simulink model "HW_1_v2_2019a_subsystem"  (R2019a)
settings: Solver=VariableStepAuto  StartTime=0.0  StopTime=70  RelTol=1e-12
model workspace (MAT data in the model file):
  d_tar = 20
values from neighbouring files (symbols this model uses):
  d_0 = 8    [acc1.m]
  t_H_tar = 1    [acc1.m]
  v_H0 = 28    [acc1.m]
  v_L0 = 36    [acc1.m]
  v_tar = 36    [acc1.m]
  x_H0 = 0    [acc1.m]
  x_L0 = 50    [acc1.m]
undefined symbols (not defined in the file or in its folder): sigbuilder_block
libraries: cstblocks x3
settings Model: Creator=jake  LastModifiedBy=andreasjonsson
settings DebuggingCC: SFMachineParentedDataDiag=error

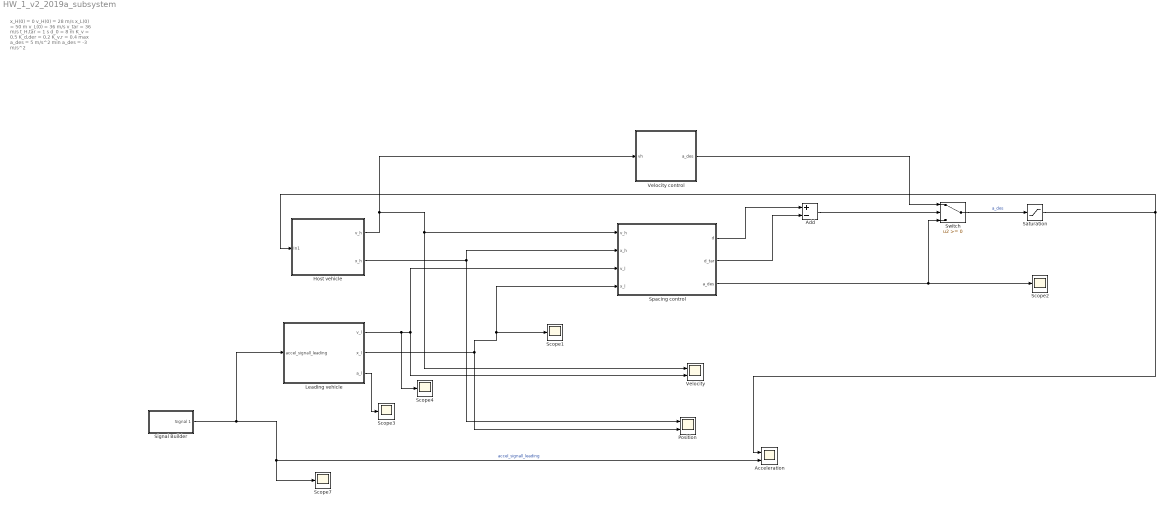
== system HW_1_v2_2019a_subsystem ==
  note: x_H(0) = 0
      | v_H(0) = 28 m/s
      |
      | x_L(0) = 50 m
      | v_L(0) = 36 m/s
      |
      | v_tar = 36 m/s
      | t_H,tar = 1 s
      | d_0 = 8 m
      |
      | K_v = 0.5
      | K_d,der = 0.2
      | K_v,r = 0.4
      |
      | max a_des = 5 m/s^2
      | min a_des = -3 m/s^2
  Acceleration : Scope  NumInputPorts=2
  Add : Sum  Inputs=+-
  Host vehicle : Subsystem
  Leading vehicle : Subsystem
  Position : Scope  NumInputPorts=2
  Saturation : Saturate  UpperLimit=5  LowerLimit=-3
  Scope{1..4,7} (5 alike) : Scope
  Signal Builder : Subsystem  Tag=STV Subsys  LoadFcn=sigbuilder_block('load');  StartFcn=sigbuilder_block('start');  StopFcn=sigbuilder_block('stop');  ClipboardFcn=sigbuilder_block('clipboard');  mask(Sigbuilder block){tuvar=[0:10]}
      mask help: Simulink:masks:SigbuilderBlock_MD
      mask init:
      | if ~strcmp(get_param(bdroot(gcbh),'SimulationStatus'),'stopped') tuvar = sigbuilder_block('maskInit'); end
      settings: CopyFcn=sigbuilder_block('copy');  DeleteFcn=sigbuilder_block('delete');  ModelCloseFcn=sigbuilder_block('modelClose');  PreSaveFcn=sigbuilder_block('preSave');  PauseFcn=sigbuilder_block('pause');  ContinueFcn=sigbuilder_block('continue');  NameChangeFcn=sigbuilder_block('namechange');  OpenFcn=sigbuilder_block('open',[553.5 167.25 843.75 498.75 ]);  CloseFcn=sigbuilder_block('close');
      mask Display: plot(0, 0, 100, 100,[2, 2, 32, 32, 2], [68, 8, 8, 68, 68],[32, 2], [38, 38], [32, 19, 2],[53, 60, 44], [32, 17, 17, 2],[16, 16, 31, 31]);txt = getActiveGroup(gcbh);text(2, 100, txt,'verticalAlignment', 'top');
  Spacing control : Subsystem
  Switch : Switch
  Velocity : Scope  NumInputPorts=2
  Velocity control : Subsystem
  wires:
  Switch/1 -> Saturation/1  "a_des"
  Signal Builder/1(Signal 1) -> Leading vehicle/1(accel_signall_leading), Scope7/1, Acceleration/2  "accel_signall_leading"
  Saturation/1 -> Host vehicle/1(In1), Acceleration/1
  Add/1 -> Switch/2
  Host vehicle/1(v_h) -> Velocity control/1(vh), Velocity/1, Spacing control/1(v_h)
  Host vehicle/2(x_h) -> Spacing control/2(x_h), Position/1
  Leading vehicle/1(v_l) -> Spacing control/3(v_l), Velocity/2, Scope4/1
  Leading vehicle/2(x_l) -> Spacing control/4(x_l), Scope1/1, Position/2
  Leading vehicle/3(a_l) -> Scope3/1
  Velocity control/1(a_des) -> Switch/1
  Spacing control/3(a_des) -> Scope2/1, Switch/3
  Spacing control/1(d) -> Add/1
  Spacing control/2(d_tar) -> Add/2

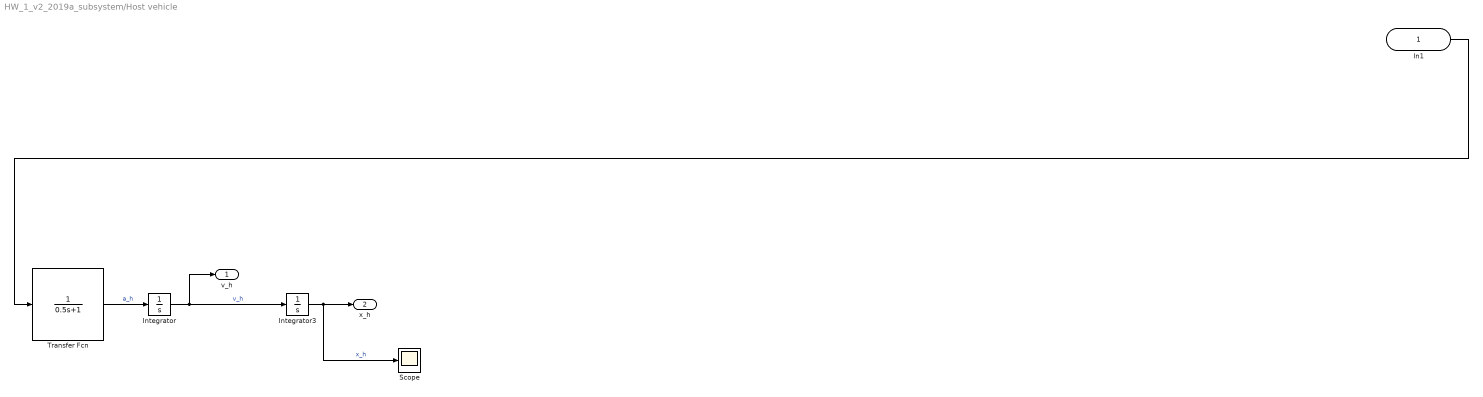
== system HW_1_v2_2019a_subsystem/Host vehicle ==
  In1 : Inport
  Integrator : Integrator  InitialCondition=v_H0
  Integrator3 : Integrator  InitialCondition=x_H0
  Scope : Scope
  Transfer Fcn : TransferFcn  Denominator=[0.5 1]
  v_h : Outport
  x_h : Outport  Port=2
  wires:
  Integrator/1 -> Integrator3/1, v_h/1  "v_h"
  Transfer Fcn/1 -> Integrator/1  "a_h"
  In1/1 -> Transfer Fcn/1
  Integrator3/1 -> Scope/1, x_h/1  "x_h"

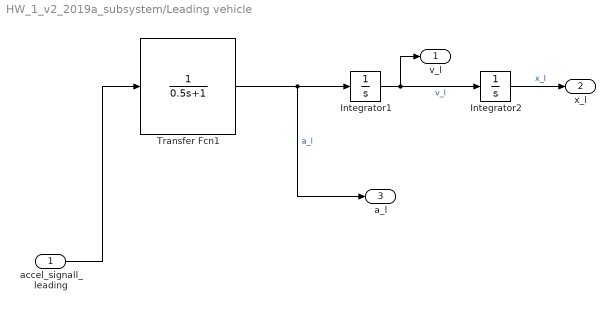
== system HW_1_v2_2019a_subsystem/Leading vehicle ==
  accel_signall_leading : Inport
  Integrator1 : Integrator  InitialCondition=v_L0
  Integrator2 : Integrator  InitialCondition=x_L0
  Transfer Fcn1 : TransferFcn  Denominator=[0.5 1]
  v_l : Outport
  x_l : Outport  Port=2
  a_l : Outport  Port=3
  wires:
  Integrator2/1 -> x_l/1  "x_l"
  accel_signall_leading/1 -> Transfer Fcn1/1
  Integrator1/1 -> Integrator2/1, v_l/1  "v_l"
  Transfer Fcn1/1 -> a_l/1, Integrator1/1  "a_l"

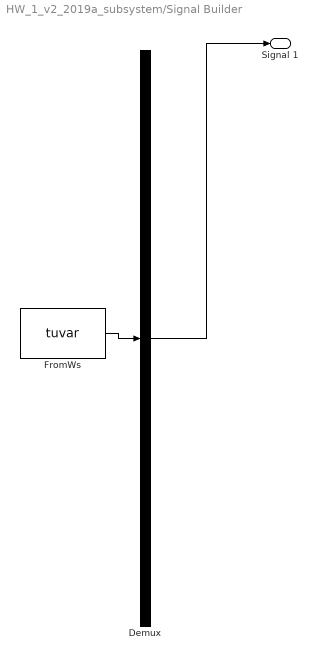
== system HW_1_v2_2019a_subsystem/Signal Builder ==
  Demux : Demux  Tag=STV Demux  Outputs=1
  FromWs : FromWorkspace  Tag=STV FromWs  VariableName=tuvar  SampleTime=0
      SigBuilderData=|
      | common.afterFinalStr = 'Extrapolate'
      | common.sampleTime = 0
      | dataSet.timeRange = [0 46]
      | dataSet.name = 'Group 1'
      | sbobj.Groups.Name = 'Group 1'
      | sbobj.Groups.Signals.Name = 'Signal 1'
      | sbobj.Groups.Signals.XData = [0 10 10.5 13.5 14 40 40.5 43.5 44 46]
      | sbobj.Groups.Signals.YData = [0 0 -2 -2 0 0 2 2 0 0.02]
      | sbobj.Groups.TimeRange = [0 46]
  Signal 1 : Outport  Tag=STV Outport  VectorParamsAs1DForOutWhenUnconnected=on
  wires:
  Demux/1 -> Signal 1/1
  FromWs/1 -> Demux/1

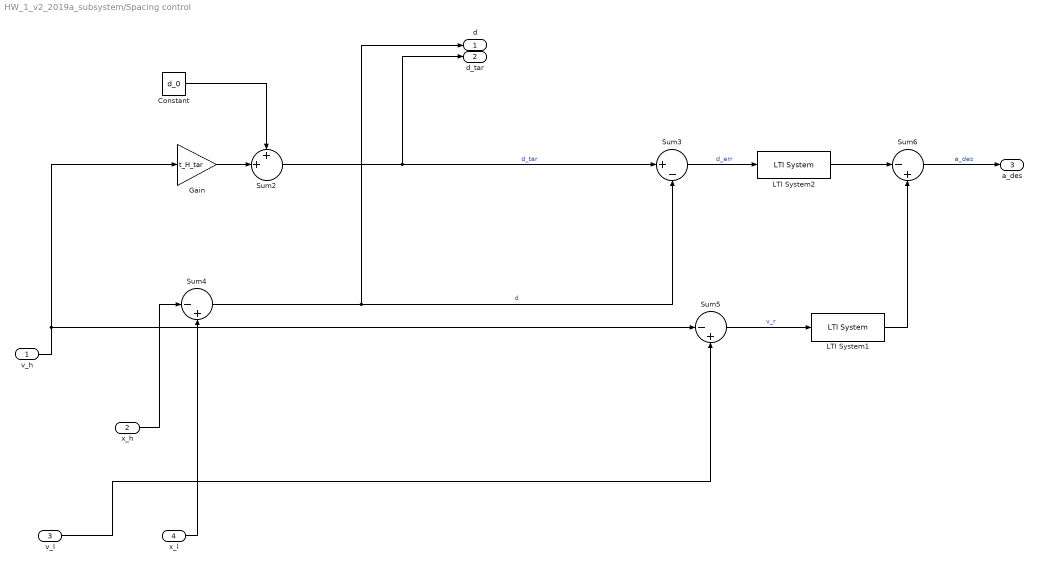
== system HW_1_v2_2019a_subsystem/Spacing control ==
  v_h : Inport
  x_h : Inport  Port=2
  v_l : Inport  Port=3
  x_l : Inport  Port=4
  Constant : Constant  Value=d_0
  Gain : Gain  Gain=t_H_tar
  LTI System1 : cstblocks/LTI System  sys=K_v_r  IC=[]
  LTI System2 : cstblocks/LTI System  sys=K_d_err  IC=[]
  Sum2 : Sum  Inputs=++|
  Sum3 : Sum  Inputs=|+-
  Sum4 : Sum  Inputs=|-+
  Sum5 : Sum  Inputs=|-+
  Sum6 : Sum  Inputs=|-+
  d : Outport
  d_tar : Outport  Port=2
  a_des : Outport  Port=3
  wires:
  x_l/1 -> Sum4/2
  v_l/1 -> Sum5/2
  Sum6/1 -> a_des/1  "a_des"
  Sum4/1 -> d/1, Sum3/2  "d"
  LTI System1/1 -> Sum6/2
  v_h/1 -> Sum5/1, Gain/1
  Gain/1 -> Sum2/2
  Sum5/1 -> LTI System1/1  "v_r"
  Sum3/1 -> LTI System2/1  "d_err"
  x_h/1 -> Sum4/1
  Sum2/1 -> d_tar/1, Sum3/1  "d_tar"
  Constant/1 -> Sum2/1
  LTI System2/1 -> Sum6/1

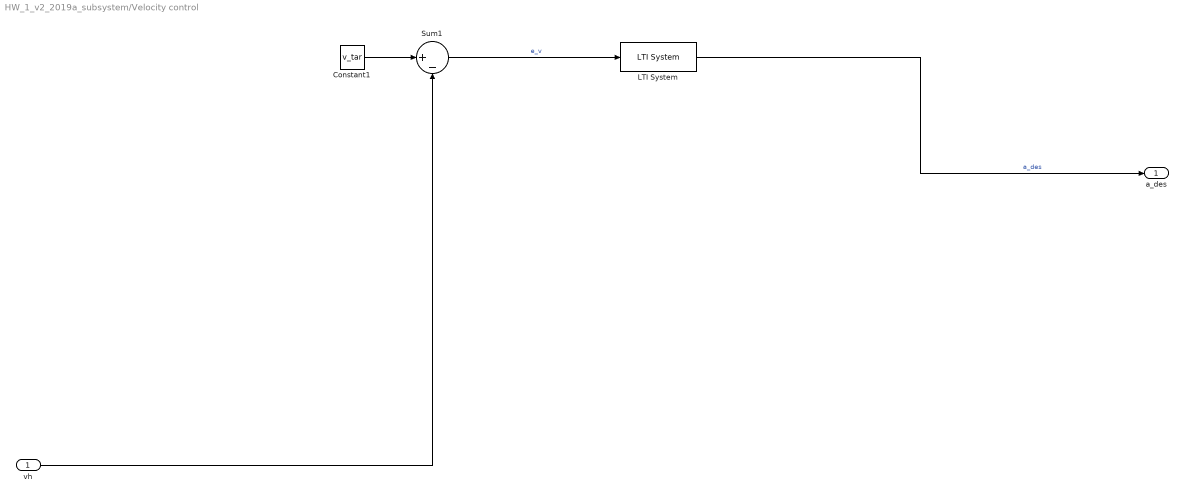
== system HW_1_v2_2019a_subsystem/Velocity control ==
  vh : Inport
  Constant1 : Constant  Value=v_tar
  LTI System : cstblocks/LTI System  sys=K_v  IC=[]
  Sum1 : Sum  Inputs=|+-
  a_des : Outport
  wires:
  LTI System/1 -> a_des/1  "a_des"
  vh/1 -> Sum1/2
  Constant1/1 -> Sum1/1
  Sum1/1 -> LTI System/1  "e_v"
